simulink subsystem "PTO_Controller_Reactive"  (R2021b)
settings: Solver=VariableStepAuto  StartTime=0.0  StopTime=10.0  RelTol=1e-3
undefined symbols (not defined in the file): wsc
settings Model: Creator=Derek  LastModifiedBy=Derek

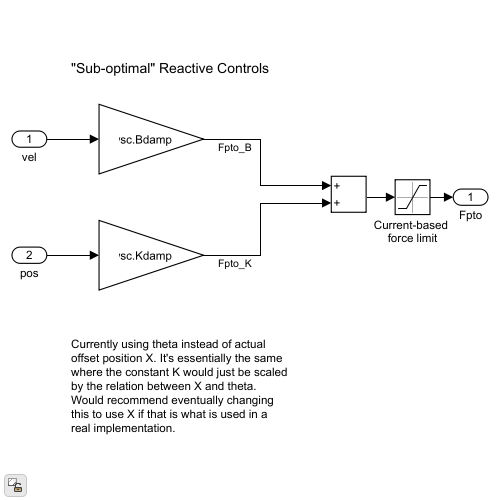
[thumbnail: Simulink's stored preview of the top-level diagram]
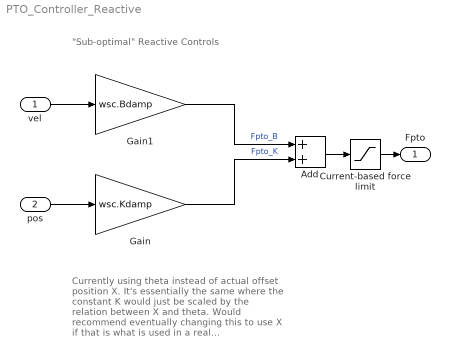
== system PTO_Controller_Reactive ==
  note: "Sub-optimal" Reactive Controls
  note: Currently using theta instead of actual offset position X. It's essentially the same where the constant K would just be scaled by the relation between X and theta. Would recommend eventually changing this to use X if that is what is used in a real implementation.
  vel : Inport
  pos : Inport  Port=2
  Add : Sum
  Current-based force limit : Saturate  UpperLimit=wsc.Fpto_lim  LowerLimit=-wsc.Fpto_lim
  Gain : Gain  Gain=wsc.Kdamp
  Gain1 : Gain  Gain=wsc.Bdamp
  Fpto : Outport
  wires:
  Gain1/1 -> Add/1  "Fpto_B"
  Gain/1 -> Add/2  "Fpto_K"
  vel/1 -> Gain1/1
  pos/1 -> Gain/1
  Add/1 -> Current-based force limit/1
  Current-based force limit/1 -> Fpto/1
